simulink model "Ass_5_ex"  (R2022a)
settings: Solver=FixedStepAuto  StartTime=0.0  StopTime=inf  FixedStep=0.2  RelTol=1e-3
settings Model: Creator=ArriGE66  LastModifiedBy=jacopo

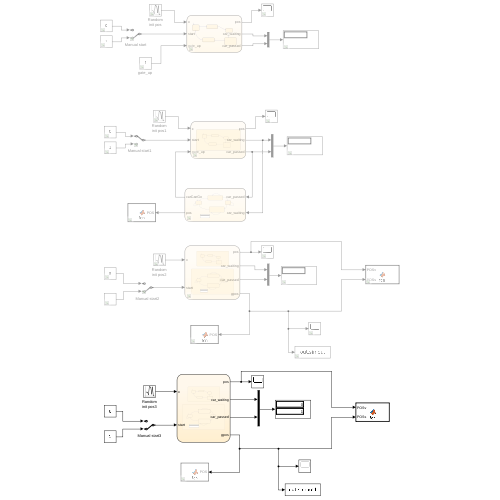
[thumbnail: Simulink's stored preview of the top-level diagram]
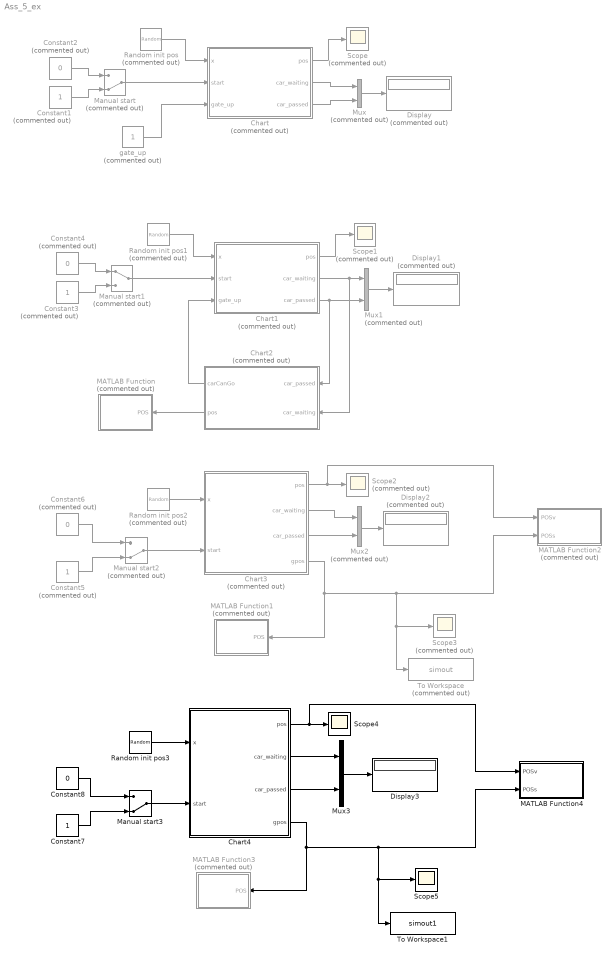
== system Ass_5_ex ==
  Chart : Stateflow chart  Commented=on  TreatAsAtomicUnit=on
  Chart1 : Stateflow chart  Commented=on  TreatAsAtomicUnit=on
  Chart2 : Stateflow chart  Commented=on  TreatAsAtomicUnit=on
  Chart3 : Stateflow chart  Commented=on  TreatAsAtomicUnit=on
  Chart4 : Stateflow chart  TreatAsAtomicUnit=on
  Constant1 : Constant  Commented=on
  Constant2 : Constant  Commented=on  Value=0
  Constant3 : Constant  Commented=on
  Constant4 : Constant  Commented=on  Value=0
  Constant5 : Constant  Commented=on
  Constant6 : Constant  Commented=on  Value=0
  Constant7 : Constant
  Constant8 : Constant  Value=0
  Display : Display  Commented=on
  Display1 : Display  Commented=on
  Display2 : Display  Commented=on
  Display3 : Display
  MATLAB Function : MATLAB Function  Commented=on  TreatAsAtomicUnit=on
  MATLAB Function1 : MATLAB Function  Commented=on  TreatAsAtomicUnit=on
  MATLAB Function2 : MATLAB Function  Commented=on  TreatAsAtomicUnit=on
  MATLAB Function3 : MATLAB Function  Commented=on  TreatAsAtomicUnit=on
  MATLAB Function4 : MATLAB Function  TreatAsAtomicUnit=on
  Manual start : ManualSwitch  Commented=on  CurrentSetting=0
  Manual start1 : ManualSwitch  Commented=on
  Manual start2 : ManualSwitch  Commented=on  CurrentSetting=0
  Manual start3 : ManualSwitch  CurrentSetting=0
  Mux : Mux  Commented=on  Inputs=2
  Mux1 : Mux  Commented=on  Inputs=2
  Mux2 : Mux  Commented=on  Inputs=2
  Mux3 : Mux  Inputs=2
  Random init pos : RandomNumber  Commented=on  Mean=-15  Variance=5
  Random init pos1 : RandomNumber  Commented=on  Mean=-15  Variance=5  SampleTime=0.2
  Random init pos2 : RandomNumber  Commented=on  Mean=-15  Variance=5  SampleTime=0.2
  Random init pos3 : RandomNumber  Mean=-15  Variance=5  SampleTime=0.2
  Scope{,1..3} (4 alike) : Scope  Commented=on
  Scope4 : Scope
  Scope5 : Scope
  To Workspace : ToWorkspace  Commented=on  VariableName=simout  SampleTime=-1
  To Workspace1 : ToWorkspace  VariableName=simout1  SampleTime=-1
  "gate_up " : Constant  Commented=on
  wires:
  Random init pos/1 -> Chart/1(x)
  Constant1/1 -> Manual start/2
  Constant2/1 -> Manual start/1
  Manual start/1 -> Chart/2(start)
  "gate_up "/1 -> Chart/3(gate_up)
  Chart/1(pos) -> Scope/1
  Mux/1 -> Display/1
  Chart/2(car_waiting) -> Mux/1
  Chart/3(car_passed) -> Mux/2
  Constant3/1 -> Manual start1/2
  Manual start1/1 -> Chart1/2(start)
  Constant4/1 -> Manual start1/1
  Chart1/1(pos) -> Scope1/1
  Random init pos1/1 -> Chart1/1(x)
  Mux1/1 -> Display1/1
  Chart1/2(car_waiting) -> Chart2/2(car_waiting), Mux1/1
  Chart1/3(car_passed) -> Chart2/1(car_passed), Mux1/2
  Chart2/1(carCanGo) -> Chart1/3(gate_up)
  Chart2/2(pos) -> MATLAB Function/1(POS)
  Chart3/1(pos) -> Scope2/1, MATLAB Function2/1(POSv)
  Manual start2/1 -> Chart3/2(start)
  Mux2/1 -> Display2/1
  Constant6/1 -> Manual start2/1
  Chart3/3(car_passed) -> Mux2/2
  Constant5/1 -> Manual start2/2
  Random init pos2/1 -> Chart3/1(x)
  Chart3/4(gpos) -> MATLAB Function1/1(POS), To Workspace/1, Scope3/1, MATLAB Function2/2(POSs)
  Chart3/2(car_waiting) -> Mux2/1
  Chart4/4(gpos) -> MATLAB Function3/1(POS), To Workspace1/1, Scope5/1, MATLAB Function4/2(POSs)
  Chart4/1(pos) -> MATLAB Function4/1(POSv), Scope4/1
  Manual start3/1 -> Chart4/2(start)
  Random init pos3/1 -> Chart4/1(x)
  Constant7/1 -> Manual start3/2
  Constant8/1 -> Manual start3/1
  Chart4/3(car_passed) -> Mux3/2
  Mux3/1 -> Display3/1
  Chart4/2(car_waiting) -> Mux3/1

== stateflow chart Ass_5_ex/Chart ==
  state idle
    init = x;
    pos = init;
    car_waiting = 0;
    car_passed = 0;
  state approaching
    pos = init + v*elapsed(sec);
  state stop
    tmp = pos;
    car_waiting = 1;
    car_passed = 0;
  state pass
    pos = tmp+v*elapsed(sec);
    car_waiting = 0;
    ex:
    pos = tmp + v*elapsed(sec);
    tmp = pos;
  state passed
    pos = tmp + v*elapsed(sec);
    car_passed = 1;
  (default) -> idle
  approaching -> stop : [pos >= 0]
  idle -> approaching : [start == 1]
  passed -> idle : [after(10, sec)]
  stop -> pass : [gate_up == 1]
  pass -> passed : [pos >= gate_end]
  data: gate_end local =3; v local double =1; pos output; car_waiting output; car_passed output; init local; x input; start input; gate_up input; tmp local

== matlab function Ass_5_ex/MATLAB Function ==
  data: POS input
function fcn(POS)

    a = 0.5;
    c = 2;
    L = 4;
    b = a + L*cos(POS);
    d = c + L*sin(POS);
    plot([a b], [c d], 'r', 'LineWidth', 2)
    hold on
    plot([0.5 0.5], [0 2], 'b', 'LineWidth', 8)
    xlim([0 6])
    ylim([0 6])
    
end

== stateflow chart Ass_5_ex/Chart3 ==
  state superstate1 [parallel]
    settings: executionOrder=1
    state idle
      init = x;
      pos = init;
      car_waiting = 0;
      car_passed = 0;
    state approaching
      pos = init + v*elapsed(sec);
    state stop
      tmp = pos;
      car_waiting = 1;
      car_passed = 0;
    state pass
      pos = tmp+v*elapsed(sec);
      car_waiting = 0;
      ex:
      pos = tmp + v*elapsed(sec);
      tmp = pos;
    state passed
      pos = tmp + v*elapsed(sec);
      car_passed = 1;
    (default) -> idle
    approaching -> stop : [pos >= 0]
    idle -> approaching : [start == 1]
    passed -> idle : [after(10, sec)]
    stop -> pass : [gate_up == 1]
    pass -> passed : [pos >= gate_end]
  state superstate2 [parallel]
    settings: executionOrder=2
    note: == 0 before
    note: probabilmente usare matlab function per
        | fare raise
        | hp per ora: raise = 1 alza, raise = 0 fermo
        | raise = - 1 abbassa
    state raising
      [gpos, gate_up] = gateAction(T, raise, gpos);
    note: gateUP viene calcolato da funzione
        | gateUP è uno se angolo è pi/2
    state up
      % gpos = pi/2;
    state down
      gpos = 0;
      gate_up = 0;
      raise = 0;
    state lowering
      [gpos, gate_up] = gateAction(T, raise, gpos);
    note: problema a scendere
    note: == 1 before
        | NaN else in function
    raising -> raising [order 1] : [gate_up > 1] {raise = 1, T = elapsed(sec)}
    raising -> up [order 2] : [gate_up == 1]
    down -> raising [order 2] : [car_waiting == 1] {raise = 1, T = elapsed(sec)}
    (default) -> down
    up -> up [order 1] : [car_passed == 0]
    down -> down [order 1] : [car_waiting == 0]
    lowering -> down [order 2] : [gate_up == 0]
    up -> lowering [order 2] : [car_passed == 1] {raise = -1, T = elapsed(sec)}
    lowering -> lowering [order 1] : [gate_up > 1] {raise = -1, T = elapsed(sec)}
  data: vpos function_output double; vgu function_output; vt function_input; vr function_input; vposin function_input; gate_end local =3; v local double =1; pos output; car_waiting output; car_passed output; init local; x input; start input; tmp local; gpos output; T local; raise local; gate_up local
  function [vpos, vgu] = gateAction(vt, vr, vposin):
    | function [vpos, vgu] = gateAction(vt, vr, vposin)
    | 
    | % vt is time
    | % vr is raise command
    | 
    | % vpos is pos
    | % vgu is gate_up
    | 
    | % gate specs
    | wmax = 4*pi/180;                                                            % rad/s, maximum angular velocity of gate
    | dwmax = 1*pi/180;                                                           % rad/s, maximum angular acceleration of gate
    | DC = 0;                                                                     % rad,   down condition
    | UC = pi/2;                                                                  % rad,   up condition
    | 
    | % perché non accelera?
    | % è giusta la legge? Io ho sempre deltaT
    | 
    | % x = k*t
    | % xb = k*t
    | % xc = k*(tb + dt)
    | % xc = xb + k*dt
    | % finché è lineare va bene
    | 
    | % ma se è quadratica
    | % x = k*t^2
    | % xb = k*tb
    | % xc = k*(tb + dt)^2
    | % xc = k*tb^2 + k*dt^2 + 2*k*tb*dt
    | % quindi, almeno ho scoperto che la legge non è giusta...
    | % adesso devo capire come considerare tb, i.e. TUTTO il tempo fino
    | % all'istante precedente
    | % variabile che è inizializzata a zero nella funzione e continua a uscire e
    | % rientrare con incremento?
    | % usare qualcosa di built-in con il tempo?
    | 
    | if vr == 1
    | %     vpos = vposin + wmax*vt + 1/2*dwmax*vt^2;
    |     vpos = vposin + 1/2*dwmax*vt^2;
    | elseif vr == - 1
    | %     vpos = UC*0 + vposin - wmax*vt - 1/2*dwmax*vt^2;
    |     vpos = UC*0 + vposin - 1/2*dwmax*vt^2;
    | else
    |     vpos = vposin;
    | end
    | 
    | if abs(vpos - DC) < 1e-2
    |     vgu = 0;
    | elseif abs(vpos - UC) < 1e-2
    |     vgu = 1;
    | else
    |     vgu = 2;
    | end
    | 
    | 
    | end

== matlab function Ass_5_ex/MATLAB Function2 ==
  data: POSv input; POSs input
function fcn(POSv, POSs)

    a = 0;
    c = 2;
    L = 4;
    b = a + L*cos(POSs);
    d = c + L*sin(POSs);
    clf
    plot3([0 0], [a b], [c d], 'r', 'LineWidth', 2)
    hold on
    plot3([0 0], [0 0], [0 2], 'b', 'LineWidth', 8)
    hold on
    plot3(POSv, 2, 0, '*k', 'LineWidth', 10)
    grid on
    xlim([-6 1])
    ylim([-0.5 6])
    zlim([0 6])
    
end

== matlab function Ass_5_ex/MATLAB Function1 ==
  data: POS input
function fcn(POS)

    a = 0.5;
    c = 2;
    L = 4;
    b = a + L*cos(POS);
    d = c + L*sin(POS);
    clf
    plot([a b], [c d], 'r', 'LineWidth', 2)
    hold on
    plot([0.5 0.5], [0 2], 'b', 'LineWidth', 8)
    xlim([0 6])
    ylim([0 6])
    
end

== stateflow chart Ass_5_ex/Chart4 ==
  state superstate1 [parallel]
    settings: executionOrder=1
    state idle
      init = x;
      pos = init;
      car_waiting = 0;
      car_passed = 0;
    state approaching
      pos = init + v*elapsed(sec);
    state stop
      tmp = pos;
      car_waiting = 1;
      car_passed = 0;
    state pass
      pos = tmp+v*elapsed(sec);
      car_waiting = 0;
      ex:
      pos = tmp + v*elapsed(sec);
      tmp = pos;
    state passed
      pos = tmp + v*elapsed(sec);
      car_passed = 1;
    (default) -> idle
    approaching -> stop : [pos >= 0]
    idle -> approaching : [start == 1]
    passed -> idle : [after(10, sec)]
    stop -> pass : [gate_up == 1]
    pass -> passed : [pos >= gate_end]
  state superstate2 [parallel]
    settings: executionOrder=2
    note: probabilmente usare matlab function per
        | fare raise
        | hp per ora: raise = 1 alza, raise = 0 fermo
        | raise = - 1 abbassa
    state raising
      [gpos, gate_up, Tc] = gateAction(T, raise, gpos, Tc, 0);
    note: gateUP viene calcolato da funzione
        | gateUP è uno se angolo è pi/2
    state up
      % gpos = pi/2;
      oldpos = gpos;
      Tc = 0;
    state down
      gpos = 0;
      gate_up = 0;
      raise = 0;
      Tc = 0;
    state lowering
      [gpos, gate_up, Tc] = gateAction(T, raise, gpos, Tc, oldpos);
    note: problema a scendere
    note: == 1 before
        | NaN else in function
    raising -> raising [order 1] : [gate_up == 0 || gate_up > 1] {raise = 1, T = elapsed(sec)}
    raising -> up [order 2] : [gate_up == 1]
    down -> raising [order 2] : [car_waiting == 1] {raise = 1, T = elapsed(sec)}
    (default) -> down
    up -> up [order 1] : [car_passed == 0]
    down -> down [order 1] : [car_waiting == 0]
    lowering -> down [order 2] : [gate_up == 0]
    up -> lowering [order 2] : [car_passed == 1] {raise = -1, T = elapsed(sec)}
    lowering -> lowering [order 1] : [gate_up > 1] {raise = -1, T = elapsed(sec)}
  data: vpos function_output double; vgu function_output; vt function_input; vr function_input; vposin function_input; Tcum function_input; t function_output; oldpos function_input; gate_end local =3; v local double =1; pos output; car_waiting output; car_passed output; init local; x input; start input; tmp local; gpos output; T local; raise local; gate_up local; Tc local; oldpos local
  function [vpos, vgu, t] = gateAction(vt, vr, vposin, Tcum, oldpos):
    | function [vpos, vgu, t] = gateAction(vt, vr, vposin, Tcum, oldpos)
    | 
    | % vt is time
    | % vr is raise command
    | 
    | % vpos is pos
    | % vgu is gate_up
    | 
    | % gate specs
    | wmax = 4*pi/180;                                                            % rad/s, maximum angular velocity of gate
    | dwmax = 1*pi/180;                                                           % rad/s, maximum angular acceleration of gate
    | DC = 0;                                                                     % rad,   down condition
    | UC = pi/2;                                                                  % rad,   up condition
    | 
    | % perché non accelera?
    | 
    | % x = k*t
    | % xb = k*t
    | % xc = k*(tb + dt)
    | % xc = xb + k*dt
    | % finché è lineare va bene
    | 
    | % ma se è quadratica
    | % x = k*t^2
    | % xb = k*tb
    | % xc = k*(tb + dt)^2
    | % xc = k*tb^2 + k*dt^2 + 2*k*tb*dt
    | % quindi, almeno ho scoperto che la legge non è giusta...
    | % adesso devo capire come considerare tb, i.e. TUTTO il tempo fino
    | % all'istante precedente
    | % variabile che è inizializzata a zero nella funzione e continua a uscire e
    | % rientrare con incremento?
    | % usare qualcosa di built-in con il tempo?
    | 
    | t = Tcum + vt;
    | 
    | if vr == 1
    | %     vpos = vposin + wmax*vt + 1/2*dwmax*vt^2;
    | %     vpos = vposin + 1/2*dwmax*vt^2;
    |     vpos = 1/2*dwmax*t^2;
    | 
    | elseif vr == - 1
    | %     vpos = UC*0 + vposin - wmax*vt - 1/2*dwmax*vt^2;
    | %     vpos = UC*0 + vposin - 1/2*dwmax*vt^2;
    |     vpos = oldpos - 1/2*dwmax*t^2;
    | 
    | else
    |     vpos = vposin;
    | end
    | 
    | if abs(vpos - DC) < 1e-2
    |     vgu = 0;
    | elseif abs(vpos - UC) < 1e-2
    |     vgu = 1;
    | else
    |     vgu = 2;
    | end
    | 
    | 
    | end

== matlab function Ass_5_ex/MATLAB Function3 ==
  data: POS input
function fcn(POS)

    a = 0.5;
    c = 2;
    L = 4;
    b = a + L*cos(POS);
    d = c + L*sin(POS);
    clf
    plot([a b], [c d], 'r', 'LineWidth', 2)
    hold on
    plot([0.5 0.5], [0 2], 'b', 'LineWidth', 8)
    xlim([0 6])
    ylim([0 6])
    
end

== matlab function Ass_5_ex/MATLAB Function4 ==
  data: POSv input; POSs input
function fcn(POSv, POSs)

    a = 0;
    c = 2;
    L = 4;
    b = a + L*cos(POSs);
    d = c + L*sin(POSs);
    clf
    plot3([0 0], [a b], [c d], 'r', 'LineWidth', 2)
    hold on
    plot3([0 0], [0 0], [0 2], 'b', 'LineWidth', 8)
    hold on
    plot3(POSv, 2, 0, '*k', 'LineWidth', 10)
    grid on
    xlim([-6 1])
    ylim([-0.5 6])
    zlim([0 6])
    
end

== stateflow chart Ass_5_ex/Chart1 ==
  state superstate1
    state idle
      init = x;
      pos = init;
      car_waiting = 0;
      car_passed = 0;
    state approaching
      pos = init + v*elapsed(sec);
    state stop
      tmp = pos;
      car_waiting = 1;
      car_passed = 0;
    state pass
      pos = tmp+v*elapsed(sec);
      car_waiting = 0;
      ex:
      pos = tmp + v*elapsed(sec);
      tmp = pos;
    state passed
      pos = tmp + v*elapsed(sec);
      car_passed = 1;
    (default) -> idle
    approaching -> stop : [pos >= 0]
    idle -> approaching : [start == 1]
    passed -> idle : [after(10, sec)]
    stop -> pass : [gate_up == 1]
    pass -> passed : [pos >= gate_end]
  data: gate_end local =3; v local double =1; pos output; car_waiting output; car_passed output; init local; x input; start input; gate_up input; tmp local

== stateflow chart Ass_5_ex/Chart2 ==
  note: probabilmente usare matlab function per
      | fare raise
      | hp per ora: raise = 1 alza, raise = 0 fermo
      | raise = - 1 abbassa
  note: gateUP viene calcolato da funzione
      | gateUP è uno se angolo è pi/2
  state raising
    carCanGo = 0;
    T = elapsed(sec);
    [pos, gate_up] = gateAction(T, raise);
  state up
    pos = pi/2;
    carCanGo = 1;
  state down
    pos = 0;
    carCanGo = 0;
  state lowering
    carCanGo = 0;
    T = elapsed(sec);
    [pos, gate_up] = gateAction(T, raise);
  raising -> raising [order 1] : [gate_up == 0] {raise = 1}
  raising -> up [order 2] : [gate_up == 1]
  down -> raising [order 2] : [car_waiting == 1] {raise = 1}
  (default) -> down
  up -> up [order 1] : [car_passed == 0]
  down -> down [order 1] : [car_waiting == 0]
  lowering -> down [order 2] : [gate_up == 0]
  up -> lowering [order 2] : [car_passed == 1] {raise = -1}
  lowering -> lowering [order 1] : [gate_up == 1] {raise = -1}
  data: vpos function_output double; vgu function_output; vt function_input; vr function_input; car_passed input; car_waiting input; carCanGo output; raise local; gate_up local; T local; pos output
  function [vpos, vgu] = gateAction(vt, vr):
    | function [vpos, vgu] = gateAction(vt, vr)
    | 
    | % v2 is car_waiting
    | % vp is car_passed
    | % vt is time
    | % vr is raise command
    | 
    | % vpos is pos
    | % vgu is gate_up
    | 
    | % gate specs
    | wmax = 4*pi/180;                                                            % rad/s, maximum angular velocity of gate
    | dwmax = 1*pi/180;                                                           % rad/s, maximum angular acceleration of gate
    | DC = 0;                                                                     % rad,   down condition
    | UC = pi/2;                                                                  % rad,   up condition
    | 
    | % in seguito aggiungere verifica su derivata di vpos (dwmax*vt) che rispetti wmax
    | 
    | 
    | if vr == 1
    |     vpos = dwmax*vt + 1/2*dwmax*vt^2; %siccome mi dà tempo passato, non c'è bisogno: togli pure vpos da input
    | elseif vr == - 1
    |     vpos = UC - dwmax*vt - 1/2*dwmax*vt^2;
    | else
    |     vpos = NaN;
    | end
    | 
    | if vpos == DC
    |     vgu = 0;
    | elseif vpos == UC
    |     vgu = 1;
    | else
    |     vgu = NaN;
    | end
    | 
    | 
    | end
